simulink model "DC_Motor_BrakeMode_WithGearbox"  (R2018a)
settings: Solver=VariableStepAuto  StartTime=0.0  StopTime=10.0  FixedStep=1e-5  RelTol=1e-3
settings Model: Creator=Thomas  LastModifiedBy=Thomas

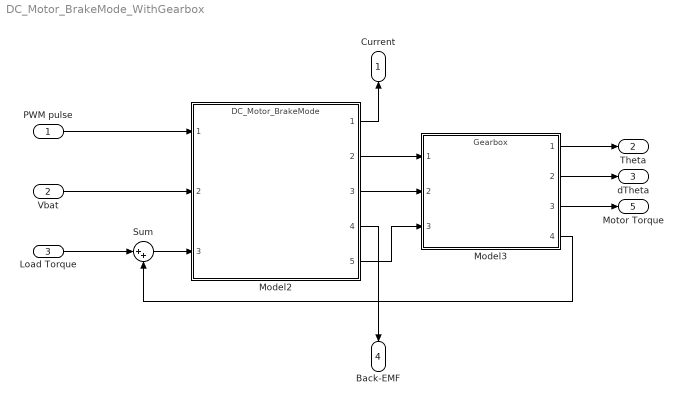
== system DC_Motor_BrakeMode_WithGearbox ==
  PWM pulse : Inport  OutDataTypeStr=int8
  Vbat : Inport  Port=2  OutDataTypeStr=double
  Load Torque : Inport  Port=3  OutDataTypeStr=double
  Model2 : ModelReference  ModelNameDialog=DC_Motor_BrakeMode  SimulationMode=Normal  ModelReferenceVersion=1.33
  Model3 : ModelReference  ModelNameDialog=Gearbox  SimulationMode=Normal  ModelReferenceVersion=1.7
  Sum : Sum  Inputs=|++
  Current : Outport
  Theta : Outport  Port=2
  dTheta : Outport  Port=3
  Back-EMF : Outport  Port=4
  Motor Torque : Outport  Port=5
  wires:
  Model2/2 -> Model3/1
  Model2/3 -> Model3/2
  Model2/1 -> Current/1
  Vbat/1 -> Model2/2
  Model3/1 -> Theta/1
  Model3/2 -> dTheta/1
  Model2/5 -> Model3/3
  Load Torque/1 -> Sum/1
  Model3/4 -> Sum/2
  Sum/1 -> Model2/3
  Model3/3 -> Motor Torque/1
  Model2/4 -> Back-EMF/1
  PWM pulse/1 -> Model2/1
